simulink model "model3"  (R2022a)
settings: Solver=VariableStepAuto  StartTime=0.0  StopTime=8  RelTol=1e-3
values from neighbouring files (symbols this model uses):
  A = [0 0 0 1 0 0; 0 0 0 0 1 0; 0 0 0 0 0 1; 0 6.5 -10 -alpha 0 0; a_51 a_52 a_53 a_54 a_55 a_56; 5 -3.6 0 0 0 -gamma]    [ME5401.m]
  B = [0 0; 0 0; 0 0; beta 11.2; b_51 b_52; 40 delta]    [ME5401.m]    (also in unity_place.m = B*q)
  C = [1 0 0 0 0 0; 0 1 0 0 0 0; 0 0 1 0 0 0]    [ME5401.m]    (also in place_pole.m = CC; unity_place.m = W_c)
  K_2 = my_lqr(A,B,Q,R)    [ME5401.m]
  L = place_pole(A',C',[-5 -10 -15 -20 -25 -30])'    [ME5401.m]
settings Model: Creator=jiaya  LastModifiedBy=jiaya
settings ModelReferenceCC: EnableRefExpFcnMdlSchedulingChecks=off
settings RTWCC: Description=Generic Real-Time Target

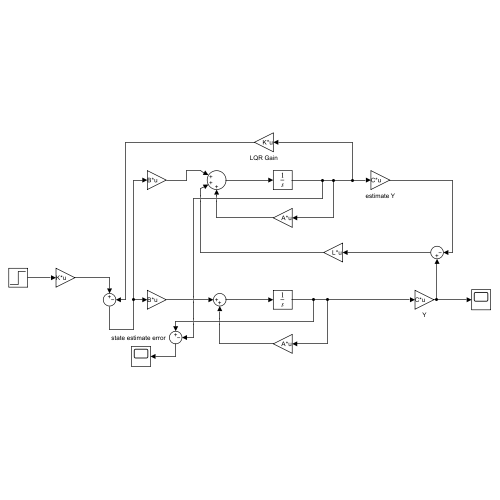
[thumbnail: Simulink's stored preview of the top-level diagram]
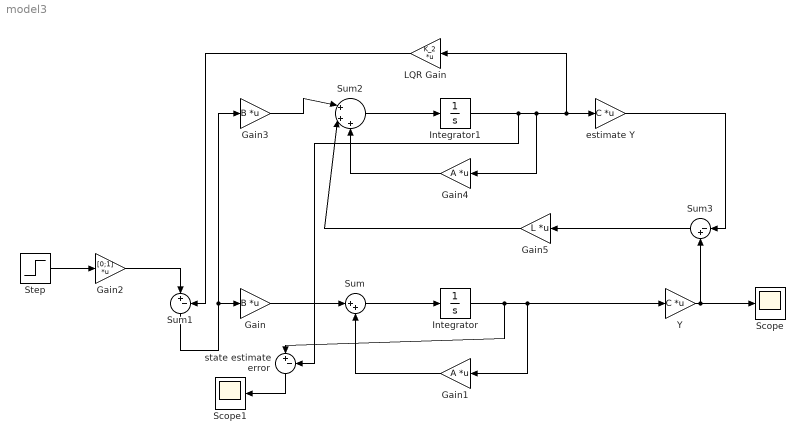
== system model3 ==
  Gain : Gain  Gain=B  Multiplication=Matrix(K*u)
  Gain1 : Gain  Gain=A  Multiplication=Matrix(K*u)
  Gain2 : Gain  Gain=[0;1]  Multiplication=Matrix(K*u)
  Gain3 : Gain  Gain=B  Multiplication=Matrix(K*u)
  Gain4 : Gain  Gain=A  Multiplication=Matrix(K*u)
  Gain5 : Gain  Gain=L  Multiplication=Matrix(K*u)
  Integrator : Integrator
  Integrator1 : Integrator
  LQR Gain : Gain  Gain=K_2  Multiplication=Matrix(K*u)
  Scope : Scope
  Scope1 : Scope
  Step : Step  Time=0  SampleTime=0
  Sum : Sum  Inputs=|++
  Sum1 : Sum  Inputs=|+-
  Sum2 : Sum  Inputs=|+++
  Sum3 : Sum  Inputs=|-+
  Y : Gain  Gain=C  Multiplication=Matrix(K*u)
  estimate Y : Gain  Gain=C  Multiplication=Matrix(K*u)
  state estimate error : Sum  Inputs=|+-
  wires:
  Gain1/1 -> Sum/2
  Gain/1 -> Sum/1
  Sum/1 -> Integrator/1
  Integrator/1 -> state estimate error/1, Y/1, Gain1/1
  Y/1 -> Scope/1, Sum3/2
  Sum1/1 -> Gain3/1, Gain/1
  Gain3/1 -> Sum2/1
  Sum2/1 -> Integrator1/1
  Integrator1/1 -> state estimate error/2, Gain4/1, LQR Gain/1, estimate Y/1
  estimate Y/1 -> Sum3/1
  Gain4/1 -> Sum2/3
  Sum3/1 -> Gain5/1
  Gain5/1 -> Sum2/2
  LQR Gain/1 -> Sum1/2
  Step/1 -> Gain2/1
  Gain2/1 -> Sum1/1
  state estimate error/1 -> Scope1/1
